simulink model "exp9"  (R2023a)
settings: Solver=VariableStepAuto  StartTime=0.0  StopTime=0.1  RelTol=1e-3
libraries: spsDiodeLib x4, spsVoltageMeasurementLib x2, spsACVoltageSourceLib x1, spsLinearTransformerLib x1, spsSeriesRLCBranchLib x1, spspowerguiLib x1
settings Model: Creator=shifa  LastModifiedBy=pc
settings DebuggingCC: UnconnectedInputMsg=warning  UnconnectedOutputMsg=warning  UnconnectedLineMsg=warning
settings ModelReferenceCC: EnableRefExpFcnMdlSchedulingChecks=on
settings RTWCC: DLArmComputeVersion=19.05

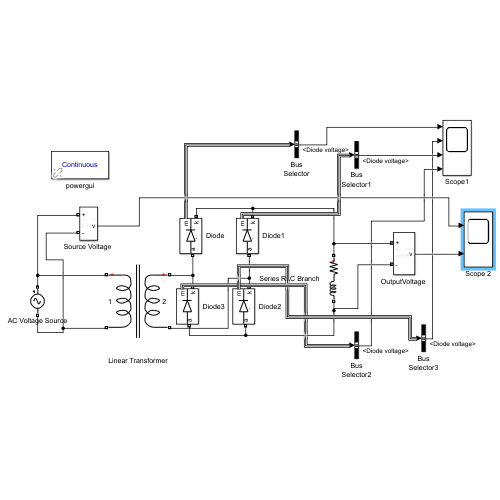
[thumbnail: Simulink's stored preview of the top-level diagram]
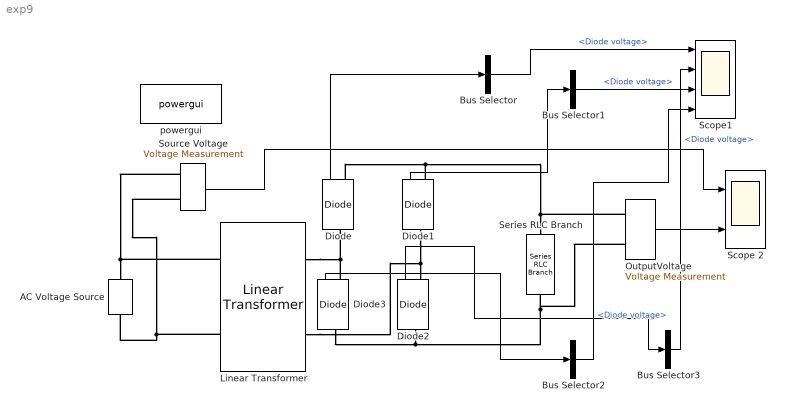
== system exp9 ==
  AC Voltage Source : spsACVoltageSourceLib/AC Voltage Source  Amplitude=230  Phase=0  Frequency=50  SampleTime=0.0001  Measurements=None  BusType=swing  Pref=10e3  Qref=0  Qmin=-inf  Qmax=+inf
  Bus Selector{,1..3} (4 alike) : BusSelector  OutputSignals=Diode voltage
  Diode{,1..3} (4 alike) : spsDiodeLib/Diode  Ron=0  Lon=0  Vf=0  IC=0  UseSnubber=0  Rs=500  Cs=0  Measurements=on
  Linear Transformer : spsLinearTransformerLib/Linear Transformer  UNITS=pu  NominalPower=[ 230e6 50 ]  winding1=[14.14 0 0]  winding2=[14.14 0 0]  ThreeWindings=off  winding3=[ 315e3 0.002 0.08 ]  RmLm=[ 500 500 ]  Measurements=None  DataType=off
  "OutputVoltage " : spsVoltageMeasurementLib/Voltage Measurement  PhasorSimulation=off  OutputType=Complex  PSBequivalent=0
  Scope 2 : Scope  NumInputPorts=2
  Scope1 : Scope  NumInputPorts=4
  Series RLC Branch : spsSeriesRLCBranchLib/Series RLC Branch  LConnTagsString=__new0  RConnTagsString=__new0  BranchType=RL  Resistance=31  Inductance=30e-3  SetiL0=off  InitialCurrent=0  Capacitance=1e-6  Setx0=off  InitialVoltage=0  Measurements=None
  "Source Voltage " : spsVoltageMeasurementLib/Voltage Measurement  PhasorSimulation=off  OutputType=Complex  PSBequivalent=0
  powergui : spspowerguiLib/powergui  Priority=1  SimulationMode=Continuous  SampleTime=50e-6  frequency=60  Iterations=50  frequencyindice=50  Pbase=100e6  ErrMax=1e-4  UnitsV=kV  UnitsW=MW  buscounter=0  FunctionMessages=off  echomessages=off  EnableUseOfTLC=off  CurrentSourceSwitches=off  DisableSnubberDevices=off  DisableRonSwitches=off  DisableVfSwitches=off  DisplayEquations=off  AutomaticDiscreteSolvers=off  SolverType=Tustin/Backward Euler (TBE)  Interpol=off  ExternalGateDelay=off  methode=off  Ts=100  x0status=blocks  SPID=on  SwTol=0  HookPort=off  NonlinearTolerance=1e-4  nMaxIteration=100  ContinueOnMaxIteration=off  RestoreLinks=warning  ResistiveCurrentMeasurement=off  Frange=[0:2:500]  Ylog=off  Xlog=on  ShowGrid=off  save=off  variable=ZData  structure=0  ZoomFFT=off  StartTime=0.0  cycles=1  DisplayStyle=1  fundamental=60  FreqAxis=off  MaxFrequency=1000  frequencyindicesteady=1  RmsSteady=1  display=off
  wires:
  "OutputVoltage "/1 -> Scope 2/2
  "Source Voltage "/1 -> Scope 2/1
  Diode/1 -> Bus Selector/1
  Diode1/1 -> Bus Selector1/1
  Diode3/1 -> Bus Selector2/1
  Diode2/1 -> Bus Selector3/1
  Bus Selector/1 -> Scope1/1  "<Diode voltage>"
  Bus Selector1/1 -> Scope1/3  "<Diode voltage>"
  Bus Selector3/1 -> Scope1/2  "<Diode voltage>"
  Bus Selector2/1 -> Scope1/4  "<Diode voltage>"
  connections:
  "Source Voltage "/LConn1 -- Linear Transformer/LConn1 -- AC Voltage Source/RConn1
  Diode/RConn1 -- Diode1/RConn1 -- "OutputVoltage "/LConn1 -- Series RLC Branch/LConn1
  Diode3/LConn1 -- Diode2/LConn1 -- "OutputVoltage "/LConn2 -- Series RLC Branch/RConn1
  "Source Voltage "/LConn2 -- Linear Transformer/LConn2 -- AC Voltage Source/LConn1
  Diode3/RConn1 -- Diode/LConn1 -- Linear Transformer/RConn1
  Diode1/LConn1 -- Linear Transformer/RConn2 -- Diode2/RConn1
